simulink model "DC_motor_gearbox"  (R2024b)
settings: Solver=ode45  StartTime=0.0  StopTime=100.0  FixedStep=0.001  RelTol=1e-3
InitFcn:
  | load_params_inertial_case
  | other_params
  | PID_calculations
values from neighbouring files (symbols this model uses):
  B_eq_model = 2.0e-6    (= 2e-06)    [load_params_inertial_case.m]    (also in other_params.m)
  J_eq_model = mot.J + mld.J/N_model^2    [other_params.m]
  K_D = K_P * T_D    [PID_calculations.m]    (also in calculations.m)
  K_I = K_P / T_I    [PID_calculations.m]    (also in calculations.m)
  K_P = DeltaK * cos(DeltaPhi)    [PID_calculations.m]    (also in calculations.m)
  N_model = 14    [other_params.m]
  rads2rpm = 60/(2*pi)    (= 9.54929658551)    [load_params_inertial_case.m]
  T_L = 1 / ((2/5) * w_gc)    [PID_calculations.m]    (also in calculations.m = 0.0633232016211)
  t_sf_model = 1.0e-2    (= 0.01)    [load_params_inertial_case.m]    (also in other_params.m)
undefined symbols (not defined in the file or in its folder): drv, mot, sens
settings Model: Creator=JS  LastModifiedBy=JS
settings SolverCC: ZeroCrossAlgorithm=Adaptive
settings DebuggingCC: IgnoredZcDiagnostic=none

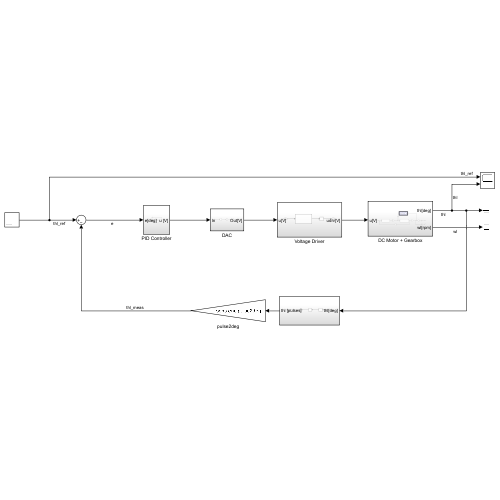
[thumbnail: Simulink's stored preview of the top-level diagram]
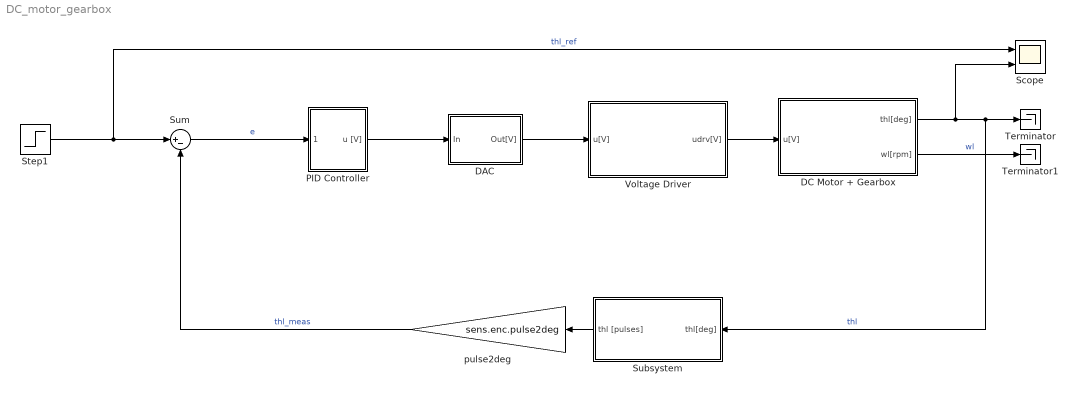
== system DC_motor_gearbox ==
  DAC : Subsystem
  DC Motor + Gearbox : Subsystem
  PID Controller : Subsystem
  Scope : Scope  NumInputPorts=2
  Step1 : Step  Time=5  After=180  SampleTime=0
  Subsystem : Subsystem
  Sum : Sum  Inputs=|+-
  Terminator : Terminator
  Terminator1 : Terminator
  Voltage Driver : Subsystem
  pulse2deg : Gain  Gain=sens.enc.pulse2deg
  wires:
  Voltage Driver/1(udrv[V]) -> DC Motor + Gearbox/1(u[V])
  DC Motor + Gearbox/1(thl[deg]) -> Scope/2, Subsystem/1(thl[deg]), Terminator/1  "thl"
  DC Motor + Gearbox/2(wl[rpm]) -> Terminator1/1  "wl"
  DAC/1(Out[V]) -> Voltage Driver/1(u[V])
  Subsystem/1(thl [pulses]) -> pulse2deg/1
  pulse2deg/1 -> Sum/2  "thl_meas"
  Sum/1 -> PID Controller/1(e[deg])  "e"
  PID Controller/1(u [V]) -> DAC/1(In)
  Step1/1 -> Scope/1, Sum/1  "thl_ref"

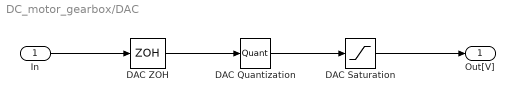
== system DC_motor_gearbox/DAC ==
  In : Inport
  DAC Quantization : Quantizer  QuantizationInterval=q_dac
  DAC Saturation : Saturate  UpperLimit=10  LowerLimit=-10
  DAC ZOH : ZeroOrderHold  SampleTime=0.001
  Out[V] : Outport
  wires:
  DAC Saturation/1 -> Out[V]/1
  In/1 -> DAC ZOH/1
  DAC ZOH/1 -> DAC Quantization/1
  DAC Quantization/1 -> DAC Saturation/1

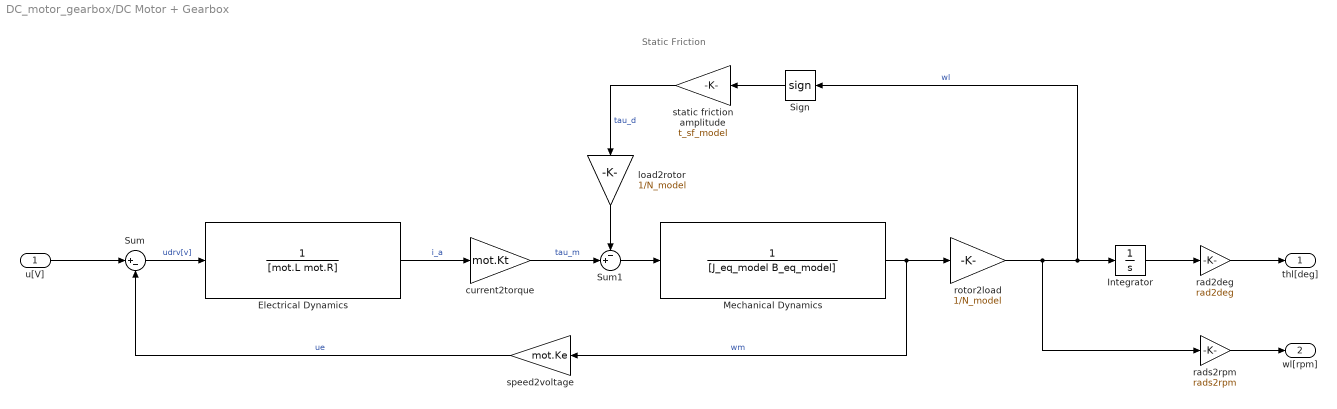
== system DC_motor_gearbox/DC Motor + Gearbox ==
  note: Static Friction
  u[V] : Inport
  Electrical Dynamics : TransferFcn  Denominator=[mot.L mot.R]
  Integrator : Integrator
  Mechanical Dynamics : TransferFcn  Denominator=[J_eq_model B_eq_model]
  Sign : Signum  ZeroCross=off
  Sum : Sum  Inputs=|+-
  Sum1 : Sum  Inputs=-+|
  current2torque : Gain  Gain=mot.Kt
  load2rotor : Gain  Gain=1/N_model
  rad2deg : Gain  Gain=rad2deg
  rads2rpm : Gain  Gain=rads2rpm
  rotor2load : Gain  Gain=1/N_model
  speed2voltage : Gain  Gain=mot.Ke
  static friction amplitude : Gain  Gain=t_sf_model
  thl[deg] : Outport
  wl[rpm] : Outport  Port=2
  wires:
  Integrator/1 -> rad2deg/1
  Mechanical Dynamics/1 -> speed2voltage/1, rotor2load/1  "wm"
  current2torque/1 -> Sum1/2  "tau_m"
  rotor2load/1 -> rads2rpm/1, Integrator/1, Sign/1  "wl"
  u[V]/1 -> Sum/1
  Electrical Dynamics/1 -> current2torque/1  "i_a"
  rad2deg/1 -> thl[deg]/1
  Sum/1 -> Electrical Dynamics/1  "udrv[v]"
  Sum1/1 -> Mechanical Dynamics/1
  rads2rpm/1 -> wl[rpm]/1
  Sign/1 -> static friction amplitude/1
  static friction amplitude/1 -> load2rotor/1  "tau_d"
  speed2voltage/1 -> Sum/2  "ue"
  load2rotor/1 -> Sum1/1

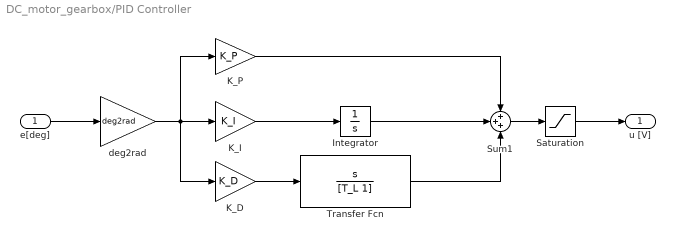
== system DC_motor_gearbox/PID Controller ==
  e[deg] : Inport
  Integrator : Integrator  ZeroCross=off
  K_D : Gain  Gain=K_D
  K_I : Gain  Gain=K_I
  K_P : Gain  Gain=K_P
  Saturation : Saturate  UpperLimit=12  LowerLimit=-12
  Sum1 : Sum  Inputs=+++
  Transfer Fcn : TransferFcn  Numerator=[1 0]  Denominator=[T_L 1]
  deg2rad : Gain  Gain=deg2rad
  u [V] : Outport
  wires:
  Sum1/1 -> Saturation/1
  deg2rad/1 -> K_P/1, K_D/1, K_I/1
  e[deg]/1 -> deg2rad/1
  K_D/1 -> Transfer Fcn/1
  Integrator/1 -> Sum1/2
  Saturation/1 -> u [V]/1
  K_I/1 -> Integrator/1
  Transfer Fcn/1 -> Sum1/3
  K_P/1 -> Sum1/1

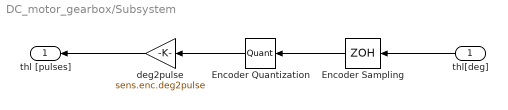
== system DC_motor_gearbox/Subsystem ==
  thl[deg] : Inport
  Encoder Quantization : Quantizer  QuantizationInterval=q_en_1
  Encoder Sampling : ZeroOrderHold  SampleTime=0.001
  deg2pulse : Gain  Gain=sens.enc.deg2pulse
  thl [pulses] : Outport
  wires:
  thl[deg]/1 -> Encoder Sampling/1
  Encoder Quantization/1 -> deg2pulse/1
  Encoder Sampling/1 -> Encoder Quantization/1
  deg2pulse/1 -> thl [pulses]/1

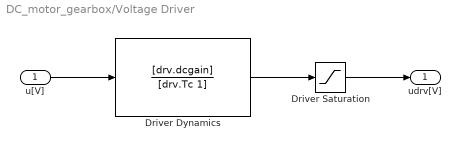
== system DC_motor_gearbox/Voltage Driver ==
  u[V] : Inport
  Driver Dynamics : TransferFcn  Numerator=[drv.dcgain]  Denominator=[drv.Tc 1]
  Driver Saturation : Saturate  UpperLimit=12  LowerLimit=-12
  udrv[V] : Outport
  wires:
  Driver Dynamics/1 -> Driver Saturation/1
  u[V]/1 -> Driver Dynamics/1
  Driver Saturation/1 -> udrv[V]/1
